simulink model "quarter_car_NL"  (R2025b)
settings: Solver=VariableStepAuto  StartTime=0.0  StopTime=10  RelTol=1e-9
values from neighbouring files (symbols this model uses):
  omega_n1 = 80    [quarter_car_parameters.m]
  tau_1 = 0.005    [quarter_car_parameters.m]
  tau_2 = 0.010    (= 0.01)    [quarter_car_parameters.m]
  tau_a = 0.025    [quarter_car_parameters.m]
  zeta_1 = 0.7    [quarter_car_parameters.m]
libraries: simulink x6
settings Model: Creator=roly2  LastModifiedBy=ettor

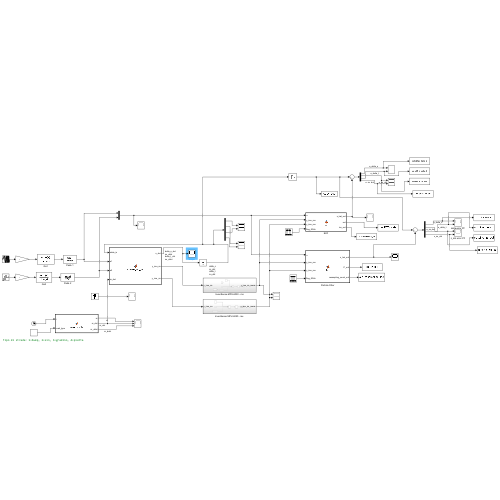
[thumbnail: Simulink's stored preview of the top-level diagram]
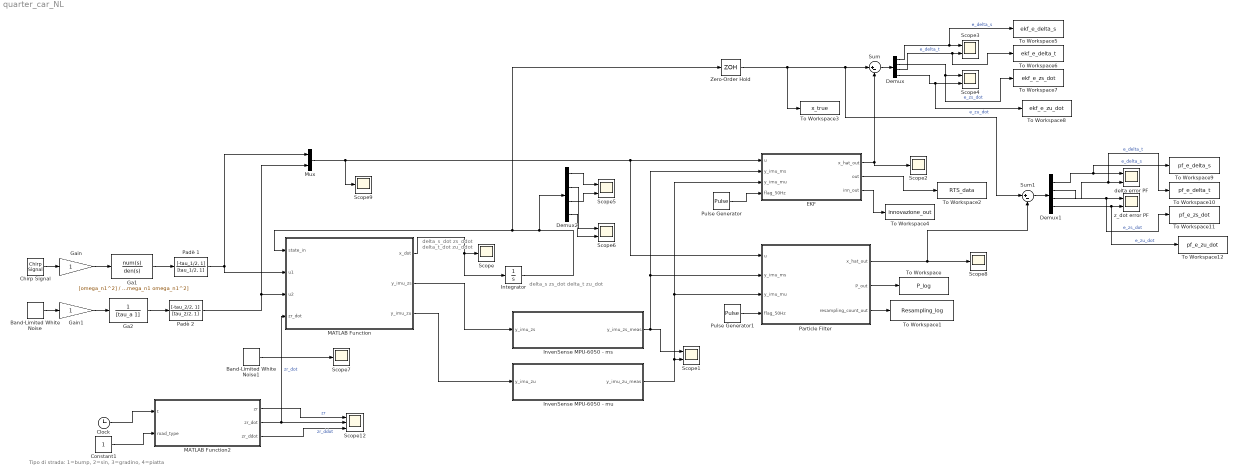
== system quarter_car_NL ==
  note: delta_s
      | zs_dot
      | delta_t
      | zu_dot
  note: delta_s_dot
      | zs_ddot
      | delta_t_dot
      | zu_ddot
  note: Tipo di strada: 1=bump, 2=sin, 3=gradino, 4=piatta
  Band-Limited White Noise : simulink/Sources/Band-Limited White Noise  Cov=[0.001]  Ts=0.1  seed=[23341]
  Band-Limited White Noise1 : simulink/Sources/Band-Limited White Noise  Cov=[0.0001]  Ts=0.01  seed=[23341]
  Chirp Signal : simulink/Sources/Chirp Signal  f1=0.1  T=20  f2=15
  Clock : Clock
  Constant1 : Constant
  Demux : Demux
  Demux1 : Demux
  Demux2 : Demux
  EKF : MATLAB Function  TreatAsAtomicUnit=on
  Ga1 : TransferFcn  Numerator=[omega_n1^2]  Denominator=[1 2*zeta_1*omega_n1 omega_n1^2]
  Ga2 : TransferFcn  Denominator=[tau_a 1]
  Gain : Gain
  Gain1 : Gain
  Integrator : Integrator  InitialCondition=[0; 0; 0; 0]
  InvenSense MPU-6050 - ms : Subsystem
  "InvenSense MPU-6050 - mu " : Subsystem
  MATLAB Function : MATLAB Function  TreatAsAtomicUnit=on
  MATLAB Function2 : MATLAB Function  TreatAsAtomicUnit=on
  Mux : Mux  Inputs=2
  Padè 1 : TransferFcn  Numerator=[-tau_1/2, 1]  Denominator=[tau_1/2, 1]
  Padè 2 : TransferFcn  Numerator=[-tau_2/2, 1]  Denominator=[tau_2/2, 1]
  Particle Filter : MATLAB Function  TreatAsAtomicUnit=on
  Pulse Generator : DiscretePulseGenerator  SampleTime=0.01
  Pulse Generator1 : DiscretePulseGenerator  SampleTime=0.01
  Scope{,2,7..9} (5 alike) : Scope
      Scope settings: ActiveDisplayYMinimum=-2.5302774552738443  ActiveDisplayYMaximum=2.9203603974718315
      Scope2 settings: ActiveDisplayYMinimum=-0.85401228792371942  ActiveDisplayYMaximum=1.07624507118322  DataLoggingVariableName=ScopeData2
      Scope7 settings: ActiveDisplayYMinimum=-0.29414404714225617  ActiveDisplayYMaximum=0.37622519846701669  DataLoggingVariableName=ScopeData7
      Scope8 settings: ActiveDisplayYMinimum=-0.19117274228267989  ActiveDisplayYMaximum=0.24070439228676016  DataLoggingVariableName=ScopeData8
      Scope9 settings: ActiveDisplayYMinimum=-1.2500782436152966  ActiveDisplayYMaximum=1.2500668722733594  DataLoggingVariableName=ScopeData10
  Scope{1,3..6} (5 alike) : Scope  NumInputPorts=2
      Scope1 settings: ActiveDisplayYMinimum=-2.689656901745356  ActiveDisplayYMaximum=2.989372585081127
      Scope3 settings: ActiveDisplayYMinimum=-0.004339833973765069  ActiveDisplayYMaximum=0.0039954664590701496  DataLoggingVariableName=ScopeData3
      Scope4 settings: ActiveDisplayYMinimum=-1.5219089390214988  ActiveDisplayYMaximum=0.83442945425216508  DataLoggingVariableName=ScopeData4
      Scope5 settings: ActiveDisplayYMinimum=-0.0322297141413675  ActiveDisplayYMaximum=0.0298789087817945  DataLoggingVariableName=ScopeData5
      Scope6 settings: ActiveDisplayYMinimum=-1  ActiveDisplayYMaximum=1  DataLoggingVariableName=ScopeData6
  Scope12 : Scope  NumInputPorts=3
      settings: ActiveDisplayYMinimum=-0.0625  ActiveDisplayYMaximum=0.0625  DataLoggingVariableName=ScopeData12
  Sum : Sum  Inputs=|+-
  Sum1 : Sum  Inputs=|+-
  To Workspace : ToWorkspace  VariableName=P_log  SampleTime=-1
  To Workspace1 : ToWorkspace  VariableName=Resampling_log  SampleTime=-1
  To Workspace10 : ToWorkspace  VariableName=pf_e_delta_t  SaveFormat=Timeseries  SampleTime=-1
  To Workspace11 : ToWorkspace  VariableName=pf_e_zs_dot  SaveFormat=Timeseries  SampleTime=-1
  To Workspace12 : ToWorkspace  VariableName=pf_e_zu_dot  SaveFormat=Timeseries  SampleTime=-1
  To Workspace2 : ToWorkspace  VariableName=RTS_data  SaveFormat=Timeseries  SampleTime=-1
  To Workspace3 : ToWorkspace  VariableName=x_true  SaveFormat=Timeseries  SampleTime=-1
  To Workspace4 : ToWorkspace  VariableName=innovazione_out  SaveFormat=Timeseries  SampleTime=-1
  To Workspace5 : ToWorkspace  VariableName=ekf_e_delta_s  SaveFormat=Timeseries  SampleTime=-1
  To Workspace6 : ToWorkspace  VariableName=ekf_e_delta_t  SaveFormat=Timeseries  SampleTime=-1
  To Workspace7 : ToWorkspace  VariableName=ekf_e_zs_dot  SaveFormat=Timeseries  SampleTime=-1
  To Workspace8 : ToWorkspace  VariableName=ekf_e_zu_dot  SaveFormat=Timeseries  SampleTime=-1
  To Workspace9 : ToWorkspace  VariableName=pf_e_delta_s  SaveFormat=Timeseries  SampleTime=-1
  Zero-Order Hold : ZeroOrderHold  SampleTime=0.01
  delta error PF : Scope  NumInputPorts=2
      settings: ActiveDisplayYMinimum=-0.0077099717145179113  ActiveDisplayYMaximum=0.0043359455767735568  DataLoggingVariableName=ScopeData11
  z_dot error PF : Scope  NumInputPorts=2
      settings: ActiveDisplayYMinimum=-0.23805957791337728  ActiveDisplayYMaximum=0.29049370002180258  DataLoggingVariableName=ScopeData9
  wires:
  MATLAB Function/1(x_dot) -> Integrator/1, Scope/1
  Integrator/1 -> Demux2/1, Zero-Order Hold/1, MATLAB Function/1(state_in)
  Ga1/1 -> Padè 1/1
  Ga2/1 -> Padè 2/1
  Chirp Signal/1 -> Gain/1
  Band-Limited White Noise/1 -> Gain1/1
  Clock/1 -> MATLAB Function2/1(t)
  Constant1/1 -> MATLAB Function2/2(road_type)
  MATLAB Function2/3(zr_ddot) -> Scope12/3  "zr_ddot"
  Gain/1 -> Ga1/1
  Gain1/1 -> Ga2/1
  Padè 1/1 -> Mux/1, MATLAB Function/2(u1)
  Padè 2/1 -> Mux/2, MATLAB Function/3(u2)
  MATLAB Function/2(y_imu_zs) -> InvenSense MPU-6050 - ms/1(y_imu_zs)
  MATLAB Function/3(y_imu_zu) -> "InvenSense MPU-6050 - mu "/1(y_imu_zu)
  InvenSense MPU-6050 - ms/1(y_imu_zs_meas) -> EKF/2(y_imu_ms), Particle Filter/2(y_imu_ms), Scope1/1
  "InvenSense MPU-6050 - mu "/1(y_imu_zu_meas) -> EKF/3(y_imu_mu), Particle Filter/3(y_imu_mu), Scope1/2
  Mux/1 -> Scope9/1, Particle Filter/1(u), EKF/1(u)
  Pulse Generator/1 -> EKF/4(flag_50Hz)
  EKF/1(x_hat_out) -> Scope2/1, Sum/2
  Sum/1 -> Demux/1
  Demux/1 -> To Workspace5/1, Scope3/1  "e_delta_s"
  Demux/2 -> To Workspace7/1, Scope4/1  "e_zs_dot"
  Demux/3 -> To Workspace6/1, Scope3/2  "e_delta_t"
  Demux/4 -> To Workspace8/1, Scope4/2  "e_zu_dot"
  Pulse Generator1/1 -> Particle Filter/4(flag_50Hz)
  Particle Filter/1(x_hat_out) -> Sum1/2, Scope8/1
  Particle Filter/2(P_out) -> To Workspace/1
  Particle Filter/3(resampling_count_out) -> To Workspace1/1
  Demux1/3 -> To Workspace10/1, delta error PF/2  "e_delta_t"
  Demux1/1 -> To Workspace9/1, delta error PF/1  "e_delta_s"
  Sum1/1 -> Demux1/1
  Demux1/2 -> To Workspace11/1, z_dot error PF/1  "e_zs_dot"
  Demux1/4 -> To Workspace12/1, z_dot error PF/2  "e_zu_dot"
  MATLAB Function2/1(zr) -> Scope12/1  "zr"
  MATLAB Function2/2(zr_dot) -> MATLAB Function/4(zr_dot), Scope12/2  "zr_dot"
  EKF/2(out) -> To Workspace2/1
  Zero-Order Hold/1 -> To Workspace3/1, Sum1/1, Sum/1
  Band-Limited White Noise1/1 -> Scope7/1
  Demux2/1 -> Scope5/1
  Demux2/3 -> Scope5/2
  Demux2/2 -> Scope6/1
  Demux2/4 -> Scope6/2
  EKF/3(inn_out) -> To Workspace4/1

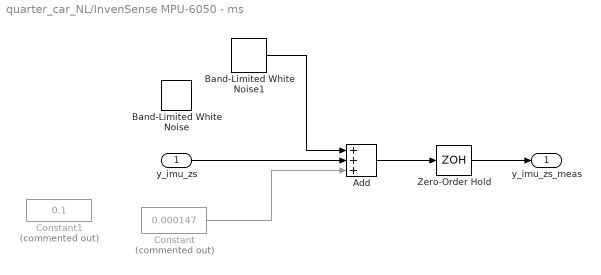
== system quarter_car_NL/InvenSense MPU-6050 - ms ==
  y_imu_zs : Inport
  Add : Sum  Inputs=+++
  Band-Limited White Noise : simulink/Sources/Band-Limited White Noise  Cov=[3.5*10^-7]  Ts=0.01  seed=[1234]
  Band-Limited White Noise1 : simulink/Sources/Band-Limited White Noise  Cov=0.0001  Ts=0.01  seed=[1234]
  Constant : Constant  Commented=on  Value=0.000147
  Constant1 : Constant  Commented=on  Value=0.1
  Zero-Order Hold : ZeroOrderHold  SampleTime=0.01
  y_imu_zs_meas : Outport
  wires:
  Add/1 -> Zero-Order Hold/1
  y_imu_zs/1 -> Add/2
  Constant/1 -> Add/3
  Zero-Order Hold/1 -> y_imu_zs_meas/1
  Band-Limited White Noise1/1 -> Add/1

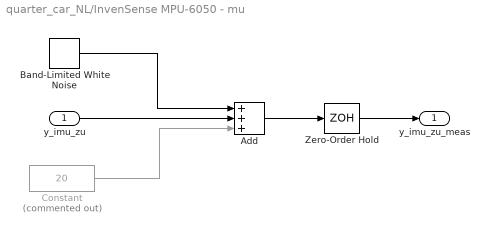
== system quarter_car_NL/InvenSense MPU-6050 - mu  ==
  y_imu_zu : Inport
  Add : Sum  Inputs=+++
  Band-Limited White Noise : simulink/Sources/Band-Limited White Noise  Cov=0.0002  Ts=0.02  seed=[23341]
  Constant : Constant  Commented=on  Value=20
  Zero-Order Hold : ZeroOrderHold  SampleTime=0.02
  y_imu_zu_meas : Outport
  wires:
  Add/1 -> Zero-Order Hold/1
  y_imu_zu/1 -> Add/2
  Constant/1 -> Add/3
  Band-Limited White Noise/1 -> Add/1
  Zero-Order Hold/1 -> y_imu_zu_meas/1

== matlab function quarter_car_NL/MATLAB Function ==
  data: state_in input; x_dot output; u1 input; u2 input; zr_dot input; parameters parameter; y_imu_zs output; y_imu_zu output
function [x_dot,y_imu_zs, y_imu_zu] = quarter_car_NL(state_in, u1, u2, zr_dot, parameters)

delta_s = state_in(1);
zs_dot = state_in(2);
delta_t = state_in(3);
zu_dot = state_in(4);

m_s = parameters.m_s+100;
m_u = parameters.m_u-10;
ks0 = parameters.ks0;
alpha = parameters.alpha;
bs = parameters.bs;
kt = parameters.kt;
bt = parameters.bt;

delta_s_dot = zs_dot - zu_dot;
delta_t_dot = zu_dot - zr_dot;

Fs = ks0 * delta_s + alpha * delta_s^3 + bs * delta_s_dot;
Ft = kt * delta_t + bt * delta_t_dot;

zs_ddot = (-Fs + u1) / m_s;
zu_ddot = (Fs - Ft - u1 + u2) / m_u;

x_dot = [delta_s_dot; zs_ddot; delta_t_dot; zu_ddot];

y_imu_zs = zs_ddot; 
y_imu_zu = zu_ddot;

== matlab function quarter_car_NL/MATLAB Function2 ==
  data: t input; zr output; zr_dot output; zr_ddot output; params parameter; road_type input
function [zr, zr_dot, zr_ddot] = road_profile(t, params, road_type)
%   road_type = 1 bump | 2 sinusoide | 3 gradino | 4 piatta

    switch road_type
        case 1  % ---- BUMP ----

            A = params.A;   % altezza [m]
            L = params.L;   % lunghezza [m]
            v = params.v;   % velocità veicolo [m/s]
            t0 = params.t0; % istante di inizio ostacolo [s]
            T = L / v;      % durata temporale bump
            
            % Il dosso inizia a t0 e finisce a t0 + T
            if t >= t0 && t <= (t0 + T)
                t_rel = t - t0; % Tempo relativo (parte da 0 quando inizia il dosso)
                phi   = 2*pi*v*t_rel / L;
                zr    = (A/2) * (1 - cos(phi));
                zr_dot   = (A*pi*v/L) * sin(phi);
                zr_ddot  = (A*2*pi^2*v^2/L^2) * cos(phi);
            else
                zr = 0;  zr_dot = 0;  zr_ddot = 0;
            end
            
        case 2  % ---- SINUSOIDE ----
            A = params.A;   % ampiezza [m]
            f = params.f;   % frequenza [Hz]
            t0 = params.t0; % istante di inizio ostacolo [s]
            
            % La strada vibra solo dopo t0
            if t >= t0
                t_rel = t - t0; % Tempo relativo
                w = 2*pi*f;
                zr   =  A * sin(w*t_rel);
                zr_dot  =  A * w * cos(w*t_rel);
                zr_ddot = -A * w^2 * sin(w*t_rel);
            else
                zr = 0;  zr_dot = 0;  zr_ddot = 0;
            end
            
        case 3  % ---- GRADINO SMUSSATO ----
            A  = params.A;    % altezza [m]
            t0 = params.t0;   % istante del gradino [s]
            tau = params.tau; % tempo di salita [s]
            
            arg  = (t - t0) / tau;
            zr   = (A/2) * (1 + tanh(arg));
            zr_dot  = (A/(2*tau)) * (sech(arg))^2;
            zr_ddot = -(A/tau^2) * (sech(arg))^2 * tanh(arg);
            
        case 4  % ---- STRADA PIATTA ----
            zr = 0;  zr_dot = 0;  zr_ddot = 0;
            
        otherwise 
            zr = 0;  zr_dot = 0;  zr_ddot = 0;
    end
end

== matlab function quarter_car_NL/EKF ==
  settings: updateMethod=DISCRETE  sampleTime=0.01
  data: u input; x_hat_out output; y_imu_ms input; y_imu_mu input; flag_50Hz input; parameters parameter; out output; inn_out output
function [x_hat_out, out , inn_out] = fcn(u, y_imu_ms , y_imu_mu, flag_50Hz, parameters)
    dt=parameters.dt_ekf;
    Q=parameters.Q;
    R_imu = parameters.R_imu;
   
    persistent x_hat P
    if isempty(x_hat)
        x_hat=[0 ; 0 ; 0; 0];   %Stato iniziale
        %P=eye(4)*0.1;            %Incertezza iniziale
        %P0_std = [0.01, 0.1, 0.002, 0.1];
        %P=eye(4).*[0.0005 , 0.005 , 0.0001 , 0.006]; %Incertezza iniziale
        P=eye(4).*[0.01, 0.1, 0.002, 0.1];
    end
    
    %% Predizione
    [x_hat_pred,P_pred, F] = predict_EKF(x_hat, P, u , parameters);
    %% Correzione
    %gestione rate diverso tra sensori
    if flag_50Hz > 0.5
        % Ciclo Pari (Pulse Alto): Abbiamo sia IMU_MS che IMU_MU
        mode = 2;
        y_meas = [y_imu_ms; y_imu_mu];
        R_curr = [R_imu, 0; 0, R_imu];
    else
        % Ciclo Dispari (Pulse Basso): Abbiamo solo l'IMU_MS
        mode = 1;
        
        y_meas = y_imu_ms;
        R_curr = R_imu;
        %Modifica: si prende sempre anche la misura di IMU_MU
        %y_meas = [y_imu_ms; y_imu_mu];
        %R_curr = [R_imu, 0; 0, R_imu*100];
    end
    
    [x_hat , P , e_out] = correct_EKF(x_hat_pred , P_pred, y_meas,R_curr,u,mode, parameters);
    x_hat_out = x_hat;
    out = [x_hat_pred, P_pred, F, x_hat , P];
    inn_out=e_out;
    
end
function [x_hat_new , P_new, F] = predict_EKF(x_hat, P, u , parameters)
    ms = parameters.m_s;    mu = parameters.m_u;
    ks0 = parameters.ks0;   kt = parameters.kt;
    bs = parameters.bs;     bt = parameters.bt;
    alpha = parameters.alpha;
    dt=parameters.dt_ekf;
    Q=parameters.Q;
    x1=x_hat(1); x2=x_hat(2) ; x3=x_hat(3) ; x4=x_hat(4);
    u1=u(1); u2=u(2);
    % Jacobiani
    A = [   0 , 1 , 0 , -1 ;
            -(ks0 + 3*alpha*x1^2)/ms , -bs/ms , 0 , bs/ms ;
            0 , 0 , 0 , 1;
            (ks0 + 3*alpha*x1^2)/mu , bs/mu , -kt/mu , -(bs+bt)/mu];
    F = eye(4) + A * dt ;
    G= [0 ; 0 ; -1 ; bt/mu];
    D=G*dt;
    
    % Predizione
    x1_dot = x2 - x4;
    x2_dot = (1/ms) * (-ks0*x1 - alpha*x1^3 - bs*(x2 - x4) + u1);
    x3_dot = x4;
    x4_dot = (1/mu) * (ks0*x1 + alpha*x1^3 + bs*(x2 - x4) - kt*x3 - bt*x4 - u1 + u2);
    x_dot = [x1_dot; x2_dot; x3_dot; x4_dot];
    x_hat_new=x_hat + x_dot * dt;
    P_new = F*P*F' + D*Q*D';
end
function [x_hat_corr , P_corr , e_out]= correct_EKF(x_hat_pred , P_pred, y_meas,R ,u, mode, parameters)
    
    ms = parameters.m_s;    mu = parameters.m_u;
    ks0 = parameters.ks0;   kt = parameters.kt;
    bs = parameters.bs;     bt = parameters.bt;
    alpha = parameters.alpha;
    x1=x_hat_pred(1); x2=x_hat_pred(2); x3=x_hat_pred(3); x4=x_hat_pred(4);
    u1=u(1); u2=u(2);
    % IMU_MS
    H1=[-(ks0 + 3*alpha*x1^2)/ms , -bs/ms , 0 , bs/ms];
    h1_exp = (1/ms) * (-ks0*x1 - alpha*x1^3 - bs*(x2-x4) + u1);
    % IMU_MU
    H2=[(ks0 + 3*alpha*x1^2)/mu , bs/mu , -kt/mu , -(bs+bt)/mu];
    h2_exp=(1/mu) * (ks0*x1 + alpha*x1^3 + bs*(x2 - x4) - kt*x3 - bt*x4 - u1 + u2);
    
    % Modifica: prendo anche vecchia misura, ma con penso diverso -> se applichi modifica decommenta questa parte
    % H=[H1 ; H2];
    % h_exp = [h1_exp ; h2_exp];
    %Se applichi modifica, commenta tutta questa parte di if and else  
    if mode==1
        %solo IMU_MS
        H=H1;
        h_exp = h1_exp;
    else
        %IMU_MS e IMU_MU
        H=[H1 ; H2];
        h_exp = [h1_exp ; h2_exp];
    end
    %Equazioni correzione
    e=y_meas-h_exp;     % Innovazione
    e_out = zeros(2,1); % Forza il vettore di uscita ad essere sempre rigorosamente 2x1
    e_out(1) = e(1);
    if mode == 2
        e_out(2) = e(2);
    end
    disp("########")
    disp(e_out);
    disp("########")
   
    S=H*P_pred*H' + R;  % Covarianza dell'innovazione
    L= P_pred*H' / S;     % Guadagno Kalman
    
    x_hat_corr=x_hat_pred + L*e;
    I=eye(4);
    P_corr=(I-L*H)*P_pred*(I-L*H)'+L*R*L';  % Forma di Joseph
    
end

== matlab function quarter_car_NL/Particle Filter ==
  settings: updateMethod=DISCRETE  sampleTime=0.01
  data: u input; x_hat_out output; y_imu_ms input; y_imu_mu input; flag_50Hz input; parameters parameter; P_out output; resampling_count_out output
function [x_hat_out , P_out, resampling_count_out] = fcn(u , y_imu_ms , y_imu_mu , flag_50Hz , parameters)
    
    dt=parameters.dt_ekf; 
    Q=parameters.Q*10; 
    N=3000; 

    threshold_n_eff=0.2; 
    epsilon_ = 0.01;

  
    persistent particles weights resampling_count

    if isempty(particles)
        %P0_variance=[0.0005, 0.005, 0.0001, 0.006]; % Incertezza Iniziale 
        %P0_variance = [0.1, 0.5, 0.05, 0.5];
        P0_variance = [0.09, 0.5, 0.05, 0.5];

        % Matrice [N x 4] per le particelle 
        particles=zeros(N,4); 
        for i=1:N
            particles(i,:)=[0 , 0 , 0 , 0]+ (P0_variance.*randn(1,4));
        end
        
        %Tutti con peso di partenza uguale 
        weights=(1/N)*ones(N,1); 

        resampling_count=0;

        
    end
    
    %% Predizione 
    [particles, weights] = predict_PF(particles, weights, Q, dt, u , parameters);
    

    %% Correzione
    %gestione rate diverso tra sensori 
    if flag_50Hz > 0.5
         % Ciclo Pari (Pulse Alto): Abbiamo sia IMU_MS che IMU_MU
        mode = 2;
    else
         % Ciclo Dispari (Pulse Basso): Abbiamo solo l'IMU_MS
        mode = 1;
    end

    [particles, weights] = correct_PF(particles, weights, y_imu_ms, y_imu_mu, u ,mode, parameters);

    %% Resampling 

    Neff = 1/sum((weights).^2);
    if (Neff/N) <= threshold_n_eff

        resampling_count = resampling_count +1; 
        disp('resampling');
        disp(resampling_count);
        disp('#############################');

        [particles, weights] = resampling_PF(particles, weights, epsilon_  ,N);
    end

    %% Out 
    [x_hat , P ]= compute_means_from_particles(particles , weights);

    x_hat_out=x_hat; 
    P_out=P; 
    resampling_count_out=resampling_count ; 


end

function [particles, weights] = predict_PF(particles, weights, Q, dt, u , parameters)
    
    ms = parameters.m_s;    mu = parameters.m_u;
    ks0 = parameters.ks0;   kt = parameters.kt;
    bs = parameters.bs;     bt = parameters.bt;
    alpha = parameters.alpha;
  
    u1=u(1); u2=u(2); 
    
    n_steps = 10; 
    dt_sim = dt / n_steps;

    Q_model_variance = [1e-6, 1e-4, 1e-6, 1e-4];
    
    for i=1:size(particles , 1)

        % Estraiamo lo stato iniziale della particella i-esima
        x1=particles(i,1); x2=particles(i,2);
        x3=particles(i,3); x4=particles(i,4);
        
        % Il rumore della strada è uno solo per l'intero passo dt
        noise_w = sqrt(Q)*randn(1); 
        
        % Ripetiamo l'integrazione 10 volte per fare 10 micro-passi
        for k = 1:n_steps
            x1_dot = x2 - x4;
            x2_dot = (1/ms) * (-ks0*x1 - alpha*x1^3 - bs*(x2 - x4) + u1);
            x3_dot = x4 - noise_w; 
            x4_dot = (1/mu) * (ks0*x1 + alpha*x1^3 + bs*(x2 - x4) - kt*x3 - bt*(x4-noise_w) - u1 + u2);
            
            % Aggiorniamo le variabili locali x1, x2, x3, x4 ad ogni micro-passo
            x1 = x1 + x1_dot * dt_sim;
            x2 = x2 + x2_dot * dt_sim;
            x3 = x3 + x3_dot * dt_sim;
            x4 = x4 + x4_dot * dt_sim;
        end
        % Solo alla fine dei 10 micro-passi salviamo il risultato finale nella matrice
        particles(i,:) = [x1, x2, x3, x4]; 
    end
end


function [particles, weights] = correct_PF(particles, weights, y_imu_ms, y_imu_mu, u ,mode, parameters)

    R_imu = parameters.R_imu;
    
    ms = parameters.m_s;    mu = parameters.m_u;
    ks0 = parameters.ks0;   kt = parameters.kt;
    bs = parameters.bs;     bt = parameters.bt;
    alpha = parameters.alpha;
    
    u1=u(1); u2=u(2); 

    likelihoods=zeros(size(particles,1),1);

    for i=1:size(particles,1)
        x1=particles(i,1); x2=particles(i,2); x3 = particles(i,3); x4=particles(i,4);

        % Misura attesa IMU_MS (Massa Sospesa)
        h_ms_exp = (1/ms) * (-ks0*x1 - alpha*x1^3 - bs*(x2-x4) + u1);  
        err_ms = y_imu_ms - h_ms_exp; 

        % Misura attesa IMU_MU (Massa Non Sospesa)
        h_mu_exp = (1/mu) * (ks0*x1 + alpha*x1^3 + bs*(x2 - x4) - kt*x3 - bt*x4 - u1 + u2);
        err_mu = y_imu_mu - h_mu_exp;

        % Calcolo Gaussiana Sensore 1
            % Se err_mu=0 restituisce 1 (il clone ha indovinato la realtà) 
            % Maggiore è err_mu più il "voto" tende a 0
        R_imu_pf = R_imu*10;    
        lik_ms = exp(-0.5 *(err_ms^2)/R_imu_pf); 

        if mode == 2
            % Sia IMU_MS che IMU_MU

            % Calcolo Gaussiana Sensore 2
            lik_mu = exp(-0.5 * (err_mu^2)/R_imu_pf); 

            % La likelihood completa 
            likelihoods(i)= lik_ms * lik_mu;
        else
            % Solo IMU_MS 
            likelihoods(i)= lik_ms; 
           
            % %Modifica: Si prende comunque anche misura Sensore 2 ma con peso minore
            %lik_mu = exp(-0.5 * (err_mu^2)/(R_imu*100)); 
            %likelihoods(i)= lik_ms * lik_mu;

        end
        
        if likelihoods(i) < 1e-100
            likelihoods(i) = 1e-100;
        end
    end
    
    % Aggiornamento pesi e normalizzazione
    weights = weights .* likelihoods;  
    weights = weights / sum(weights);  
end


function [particles_out, weights_out] = resampling_PF(particles, weights, epsilon_  ,N)

    % Ricampionamento: " il nuovo campione x_j assume il vecchio valore x_i con probabilità w_i "
    s=cumsum(weights); 
    particles_out=zeros(N,4); 

 
    scale = [0.01, 0.1, 0.005, 0.1]; % Scala basata sulle ampiezze degli stati


    for j = 1:N
        u_rand=rand(1); % Estrae numero casuale in [0,1]
        i=find(s >= u_rand , 1 ,'first'); %Trova la particella vincente

        % aggiunta piccolo disturbo
        %csi = epsilon_*randn(1,4); 
        csi = (scale .* randn(1,4)) * epsilon_;
        particles_out(j,:)=particles(i,:) + csi; 
    end
    
    % Tutti i pesi riportati a 1
    weights_out=(1/N)*ones(N,1);

end

function [x_mean , P_conv ]= compute_means_from_particles(particles , weights)
    % Media pesata 

    x_mean=particles'*weights;

    P_conv=zeros(4,4); 

    for i=1:size(particles ,1)
        x_i=particles(i,:)';
        err=x_i-x_mean;
        P_conv=P_conv + weights(i)*(err*err');
    end

end
